simulink model "bai31111"  (R2022b)
settings: Solver=ode4  StartTime=0.0  StopTime=20  FixedStep=0.0001  RelTol=1e-8
undefined symbols (not defined in the file or in its folder): k
settings Model: Creator=ASUS  LastModifiedBy=ASUS

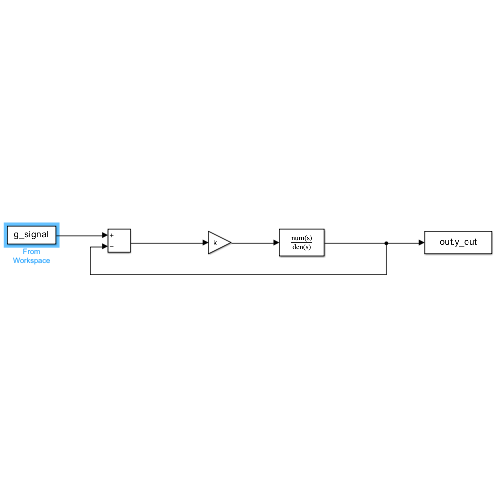
[thumbnail: Simulink's stored preview of the top-level diagram]
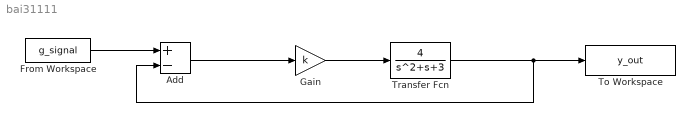
== system bai31111 ==
  Add : Sum  Inputs=+-
  From Workspace : FromWorkspace  VariableName=g_signal
  Gain : Gain  Gain=k
  To Workspace : ToWorkspace  VariableName=y_out  SaveFormat=Structure With Time  SampleTime=-1
  Transfer Fcn : TransferFcn  Numerator=[4]  Denominator=[1 1 3]
  wires:
  From Workspace/1 -> Add/1
  Add/1 -> Gain/1
  Gain/1 -> Transfer Fcn/1
  Transfer Fcn/1 -> To Workspace/1, Add/2
